simulink model "ES011A_DualEcuIdn"  (R2013b)
settings: Solver=FixedStepDiscrete  SolverMode=SingleTasking  StartTime=0.0  StopTime=1  FixedStep=0.002  RelTol=1e-3
values from neighbouring files (symbols this model uses):
  ECUCOMTIOUTFLT_CNT_U08 = DataDict.Constant    [ES011A_DualEcuIdn_DataDict.m]
  ECUID1_CNT_U08 = DataDict.Constant    [ES011A_DualEcuIdn_DataDict.m]
  ECUID2_CNT_U08 = DataDict.Constant    [ES011A_DualEcuIdn_DataDict.m]
  ECUIDINVLD_CNT_U08 = DataDict.Constant    [ES011A_DualEcuIdn_DataDict.m]
  IDENTCLECUIDNFLT_CNT_U08 = DataDict.Constant    [ES011A_DualEcuIdn_DataDict.m]
  IMCARBN_DUALECUIDNSECDRYECUIDN_CNT_U16 = DataDict.Constant    [ES011A_DualEcuIdn_DataDict.m]
  PRIMECUIDNOTREADFLT_CNT_U08 = DataDict.Constant    [ES011A_DualEcuIdn_DataDict.m]
  PRIMECUINVLDIDFLT_CNT_U08 = DataDict.Constant    [ES011A_DualEcuIdn_DataDict.m]
  SECDRYECUIDNOTREADFLT_CNT_U08 = DataDict.Constant    [ES011A_DualEcuIdn_DataDict.m]
  SECDRYECUIDNREQTIOUTVAL_CNT_U08 = DataDict.Constant    [ES011A_DualEcuIdn_DataDict.m]
  SECDRYECUINVLDIDFLT_CNT_U08 = DataDict.Constant    [ES011A_DualEcuIdn_DataDict.m]
  SECDRYECUREQIDTIOUTFLT_CNT_U08 = DataDict.Constant    [ES011A_DualEcuIdn_DataDict.m]
  VLDECUID_CNT_U08 = DataDict.Constant    [ES011A_DualEcuIdn_DataDict.m]
undefined symbols (not defined in the file or in its folder): NtcNr1, NtcSts1, sigbuilder_block
libraries: simulink x2
(part 1 of 2)
settings Model: Creator=cz68ds  LastModifiedBy=nzg49t
settings SolverCC: AutoInsertRateTranBlk=on  InsertRTBMode=Always
settings DataIOCC: LimitDataPoints=off  SaveFormat=Structure  ReturnWorkspaceOutputs=on
settings OptimizationCC: BlockReduction=off  InlineParams=on  ZeroExternalMemoryAtStartup=off  ZeroInternalMemoryAtStartup=off  OptimizeModelRefInitCode=on  LifeSpan=1
settings DebuggingCC: SignalInfNanChecking=error  SignalRangeChecking=warning  UnderspecifiedInitializationDetection=Simplified  SolverPrmCheckMsg=error  InheritedTsInSrcMsg=error  DiscreteInheritContinuousMsg=error  SingleTaskRateTransMsg=error  TasksWithSamePriorityMsg=error  SigSpecEnsureSampleTimeMsg=error  CheckMatrixSingularityMsg=error  ParameterUnderflowMsg=error  ParameterPrecisionLossMsg=error  ParameterTunabilityLossMsg=error  FixptConstUnderflowMsg=warning  FixptConstOverflowMsg=warning  VectorMatrixConversionMsg=error  SignalLabelMismatchMsg=error  UnconnectedInputMsg=error  UnconnectedOutputMsg=error  UnconnectedLineMsg=error  SFcnCompatibilityMsg=error  UniqueDataStoreMsg=warning  BusObjectLabelMismatch=error  RootOutportRequireBusObject=error  AssertControl=DisableAll  ModelReferenceIOMsg=error  ModelReferenceVersionMismatchMessage=warning  ModelReferenceIOMismatchMessage=error  ModelReferenceCSMismatchMessage=warning  ModelReferenceDataLoggingMessage=error  StateNameClashWarn=warning  StrictBusMsg=ErrorOnBusTreatedAsVector  NonBusSignalsTreatedAsBus=error  SFUnexpectedBacktrackingDiag=error  SFInvalidInputDataAccessInChartInitDiag=error  SFNoUnconditionalDefaultTransitionDiag=error  SFTransitionOutsideNaturalParentDiag=error  SFUnconditionalTransitionShadowingDiag=error  SFUndirectedBroadcastEventsDiag=error
settings ModelReferenceCC: ModelReferenceNumInstancesAllowed=Single
settings RTWCC: SystemTargetFile=autosar.tlc  GenCodeOnly=on  TemplateMakefile=ert_default_tmf  Description=AUTOSAR  GenerateReport=on  ProcessScript=autosar_make_rtw_hook  LaunchReport=on
settings CodeAppCC: GenerateComments=off  IgnoreCustomStorageClasses=off  CustomSymbolStrType=$N$R$M  CustomSymbolStrBlkIO=$N$M  SimulinkBlockComments=off
settings STFCustomTargetCC: ParMdlRefBuildCompliant=on  CompOptLevelCompliant=on  IncludeMdlTerminateFcn=off  CombineOutputUpdateFcns=on  SuppressErrorStatus=on  ERTFirstTimeCompliant=on  ERTCustomFileBanners=on  SupportNonFinite=off  SupportComplex=off  SupportContinuousTime=off  SupportNonInlinedSFcns=off  MATLABClassNameForMDSCustomization=Simulink.SoftwareTarget.ERTCustomization  AutosarCompliant=on  GRTInterface=off  SystemTargetFile=autosar.tlc
settings ERTTargetCC: CodeReplacementLibrary=ANSI_C  ConcurrentExecutionCompliant=off  IncludeMdlTerminateFcn=off  SuppressErrorStatus=on  SupportNonFinite=off  SupportComplex=off  ModelStepFunctionPrototypeControlCompliant=off  CPPClassGenCompliant=off  AutosarCompliant=on  InlinedParameterPlacement=NonHierarchical  ERTCustomFileTemplate=example_file_process.tlc  EnableUserReplacementTypes=on

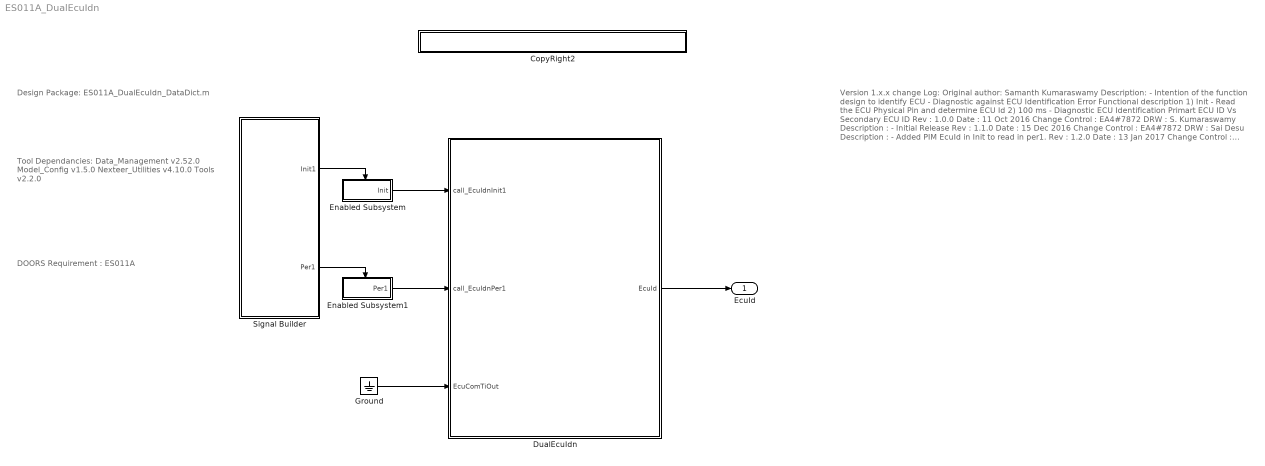
== system ES011A_DualEcuIdn ==
  note: Design Package:
      |
      | ES011A_DualEcuIdn_DataDict.m
  note: Tool Dependancies:
      |
      | Data_Management v2.52.0
      | Model_Config v1.5.0
      | Nexteer_Utilities v4.10.0
      | Tools v2.2.0
  note: DOORS Requirement :
      |
      | ES011A
  note: Version 1.x.x change Log:
      |
      | Original author: Samanth Kumaraswamy
      | Description:
      | - Intention of the function design to identify ECU
      | - Diagnostic against ECU Identification Error
      |
      | Functional description
      | 1) Init - Read the ECU Physical Pin and determine ECU Id
      | 2) 100 ms - Diagnostic ECU Identification Primart ECU ID Vs Secondary ECU ID
      |
      | Rev					: 1.0.0
      | Date					: 11 Oct 2016
      | Change Control		: EA4#7872
      | DRW					: S. Kumaraswamy
      | Description			:
      | - Initial Release
      |
      | Rev					: 1.1.0
      | Date					: 15 Dec 2016
      | Change Control		: EA4#7872
      | DRW					: Sai Desu
      | Description			:
      | - Added PIM EcuId in Init to read in per1.
      |
      | Rev					: 1.2.0
      | Date					: 13 Jan 2017
      | Change Control		: EA4#9279
      | DRW					: S. Kumaraswamy
      | Description			:
      | - Edited the PIM's name
      | - Added SetNtcSts in .m file as client call
  CopyRight2 : Subsystem  Description=|  mask(Copyright Information){none=on}
      | Copyright info block.                                               
      |                                                                     
      | Place copyright information at the top of every subsystem in design.
      mask prompts: none "No parameters"
      mask help: Place copyright information at the top of every subsystem in design.
      mask Display:
      | NxtrConf = 'Nexteer Confidential';
      | 
      | sys = bdroot; %handle for the current model ("system")
      | first = get_param(sys,'Created');
      | first = first(end-3:end);  %year is last four digits
      | 
      | last = get_param(sys,'LastModifiedDate');
      | if isempty(last)
      |     last = datestr(now,'yyyy');
      | else
      |     last = last(end-3:end);
      | end
      | 
      | if strcmp(first,last)
      |     fprintf('%s -- Copyright %s Nexteer',NxtrConf,first)
      | else
      |     fprintf('%s -- %s%s- %s Nexteer',NxtrConf,char(169),first,last)
      | end
  DualEcuIdn : Subsystem
  Enabled Subsystem : Subsystem  TreatAsAtomicUnit=on
  Enabled Subsystem1 : Subsystem  TreatAsAtomicUnit=on
  Ground : Ground
  Signal Builder : Subsystem  Tag=STV Subsys  LoadFcn=sigbuilder_block('load');  StartFcn=sigbuilder_block('start');  StopFcn=sigbuilder_block('stop');  ClipboardFcn=sigbuilder_block('clipboard');  mask(Sigbuilder block){}
      mask help: Simulink:masks:SigbuilderBlock_MD
      mask init:
      | if ~strcmp(get_param(bdroot(gcbh),'SimulationStatus'),'stopped') tuvar = sigbuilder_block('maskInit'); end
      settings: CopyFcn=sigbuilder_block('copy');  DeleteFcn=sigbuilder_block('delete');  ModelCloseFcn=sigbuilder_block('modelClose');  PreSaveFcn=sigbuilder_block('preSave');  PauseFcn=sigbuilder_block('pause');  ContinueFcn=sigbuilder_block('continue');  NameChangeFcn=sigbuilder_block('namechange');  OpenFcn=sigbuilder_block('open',[0 29.7931 1191.72 587.172 ]);  CloseFcn=sigbuilder_block('close');
      mask Display: plot(0, 0, 100, 100,[2, 2, 32, 32, 2], [68, 8, 8, 68, 68],[32, 2], [38, 38], [32, 19, 2],[53, 60, 44], [32, 17, 17, 2],[16, 16, 31, 31]);txt = getActiveGroup(gcbh);text(2, 100, txt,'verticalAlignment', 'top');
  EcuId : Outport
  wires:
  DualEcuIdn/1(EcuId) -> EcuId/1
  Enabled Subsystem/1(Init) -> DualEcuIdn/1(call_EcuIdnInit1)
  Ground/1 -> DualEcuIdn/3(EcuComTiOut)
  Signal Builder/1(Init1) -> Enabled Subsystem/Enable
  Enabled Subsystem1/1(Per1) -> DualEcuIdn/2(call_EcuIdnPer1)
  Signal Builder/2(Per1) -> Enabled Subsystem1/Enable

== system ES011A_DualEcuIdn/CopyRight2 ==

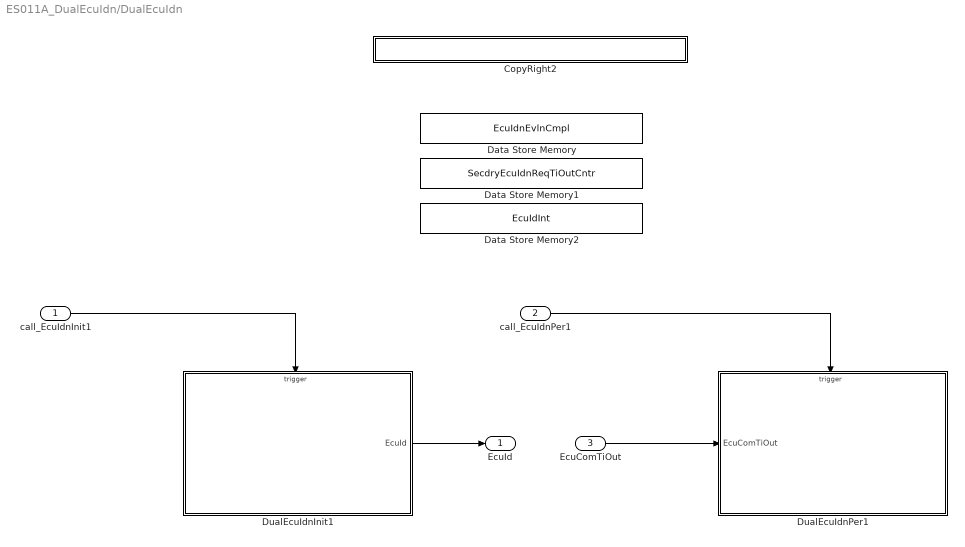
== system ES011A_DualEcuIdn/DualEcuIdn ==
  call_EcuIdnInit1 : Inport
  call_EcuIdnPer1 : Inport  Port=2
  EcuComTiOut : Inport  RequirementInfo={'linktype_rmi_doors' '00011b56 (/ESG Group/FDD Module Requirements/EA4 Specific/ES011A_DualEcuIdn)' '#ES011A_30' 'true' 'REQ:ES011A_30' '' } %GIDa_989c1e84_47d6_4077_a2ae_3e146373df7e  Port=3
  CopyRight2 : Subsystem  Description=|  mask(Copyright Information){none=on}
      | Copyright info block.                                               
      |                                                                     
      | Place copyright information at the top of every subsystem in design.
      mask prompts: none "No parameters"
      mask help: Place copyright information at the top of every subsystem in design.
      mask Display:
      | NxtrConf = 'Nexteer Confidential';
      | 
      | sys = bdroot; %handle for the current model ("system")
      | first = get_param(sys,'Created');
      | first = first(end-3:end);  %year is last four digits
      | 
      | last = get_param(sys,'LastModifiedDate');
      | if isempty(last)
      |     last = datestr(now,'yyyy');
      | else
      |     last = last(end-3:end);
      | end
      | 
      | if strcmp(first,last)
      |     fprintf('%s -- Copyright %s Nexteer',NxtrConf,first)
      | else
      |     fprintf('%s -- %s%s- %s Nexteer',NxtrConf,char(169),first,last)
      | end
  Data Store Memory : DataStoreMemory  DataStoreName=EcuIdnEvlnCmpl  OutDataTypeStr=boolean  StateMustResolveToSignalObject=on
  Data Store Memory1 : DataStoreMemory  DataStoreName=SecdryEcuIdnReqTiOutCntr  ReadBeforeWriteMsg=warning  WriteAfterWriteMsg=warning  WriteAfterReadMsg=warning  OutDataTypeStr=uint8  StateMustResolveToSignalObject=on
  Data Store Memory2 : DataStoreMemory  DataStoreName=EcuIdInt  OutDataTypeStr=uint8  StateMustResolveToSignalObject=on
  DualEcuIdnInit1 : Subsystem  RequirementInfo={'linktype_rmi_doors' '00011b56 (/ESG Group/FDD Module Requirements/EA4 Specific/ES011A_DualEcuIdn)' '#ES011A_56' 'true' 'REQ:ES011A_56' '' } %GIDa_248ec188_8c94_4ea4_99f3_45ec3f411dd5  TreatAsAtomicUnit=on
  DualEcuIdnPer1 : Subsystem  TreatAsAtomicUnit=on
  EcuId : Outport  RequirementInfo={'linktype_rmi_doors' '00011b56 (/ESG Group/FDD Module Requirements/EA4 Specific/ES011A_DualEcuIdn)' '#ES011A_31' 'true' 'REQ:ES011A_31' '' } %GIDa_18f308b4_0b0b_460d_b1e9_0f3a9849a141
  wires:
  call_EcuIdnInit1/1 -> DualEcuIdnInit1/Trigger
  call_EcuIdnPer1/1 -> DualEcuIdnPer1/Trigger
  DualEcuIdnInit1/1(EcuId) -> EcuId/1
  EcuComTiOut/1 -> DualEcuIdnPer1/1(EcuComTiOut)

== system ES011A_DualEcuIdn/Enabled Subsystem ==
  Enable : EnablePort
  Function Call Trigger2 : simulink/Ports & Subsystems/Function-Call Generator  RequirementInfo={} %GIDa_b8285886_6bd1_4885_ac08_252502d484ae  sample_time=0.1  numberOfIterations=1
      settings: AttributesFormatString=%<sample_time>
  Init : Outport
  wires:
  Function Call Trigger2/1 -> Init/1

== system ES011A_DualEcuIdn/Enabled Subsystem1 ==
  Enable : EnablePort
  Function Call Trigger1 : simulink/Ports & Subsystems/Function-Call Generator  RequirementInfo={} %GIDa_41275702_d4e5_428b_b5a8_ee66f9a793ef  sample_time=0.1  numberOfIterations=1
      settings: AttributesFormatString=%<sample_time>
  Per1 : Outport
  wires:
  Function Call Trigger1/1 -> Per1/1

== system ES011A_DualEcuIdn/Signal Builder ==
  Demux : Demux  Tag=STV Demux  Outputs=2
  FromWs : FromWorkspace  Tag=STV FromWs  VariableName=tuvar  SampleTime=0
      SigBuilderData=|
      | common.afterFinalStr = 'Extrapolate'
      | common.sampleTime = 0
      | dataSet.timeRange = [0 10]
      | dataSet.name = 'Group 1'
      | sbobj.Groups.Name = 'Group 1'
      | sbobj.Groups.Signals(1).Name = 'Init1'
      | sbobj.Groups.Signals(1).XData = [0 0.1 0.1 10]
      | sbobj.Groups.Signals(1).YData = [1 1 0 0]
      | sbobj.Groups.Signals(2).Name = 'Per1'
      | sbobj.Groups.Signals(2).XData = [0 0.1 0.1 10]
      | sbobj.Groups.Signals(2).YData = [0 0 1 1]
  Init1 : Outport  Tag=STV Outport
  Per1 : Outport  Tag=STV Outport  Port=2
  wires:
  Demux/1 -> Init1/1
  FromWs/1 -> Demux/1
  Demux/2 -> Per1/1

== system ES011A_DualEcuIdn/DualEcuIdn/CopyRight2 ==

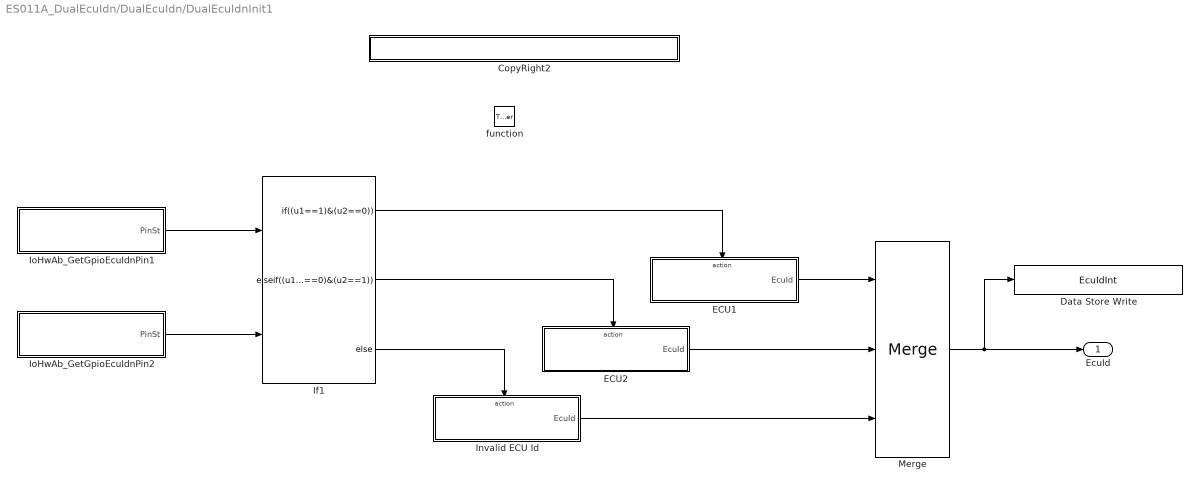
== system ES011A_DualEcuIdn/DualEcuIdn/DualEcuIdnInit1 ==
  function : TriggerPort  TriggerType=function-call
  CopyRight2 : Subsystem  Description=|  mask(Copyright Information){none=on}
      | Copyright info block.                                               
      |                                                                     
      | Place copyright information at the top of every subsystem in design.
      mask prompts: none "No parameters"
      mask help: Place copyright information at the top of every subsystem in design.
      mask Display:
      | NxtrConf = 'Nexteer Confidential';
      | 
      | sys = bdroot; %handle for the current model ("system")
      | first = get_param(sys,'Created');
      | first = first(end-3:end);  %year is last four digits
      | 
      | last = get_param(sys,'LastModifiedDate');
      | if isempty(last)
      |     last = datestr(now,'yyyy');
      | else
      |     last = last(end-3:end);
      | end
      | 
      | if strcmp(first,last)
      |     fprintf('%s -- Copyright %s Nexteer',NxtrConf,first)
      | else
      |     fprintf('%s -- %s%s- %s Nexteer',NxtrConf,char(169),first,last)
      | end
  Data Store Write : DataStoreWrite  DataStoreName=EcuIdInt
  ECU1 : Subsystem  TreatAsAtomicUnit=on
  ECU2 : Subsystem  TreatAsAtomicUnit=on
  If1 : If  NumInputs=2  IfExpression=(u1==1)&(u2==0)  ElseIfExpressions=(u1==0)&(u2==1)
  Invalid ECU Id : Subsystem  TreatAsAtomicUnit=on
  IoHwAb_GetGpioEcuIdnPin1 : Subsystem
  IoHwAb_GetGpioEcuIdnPin2 : Subsystem
  Merge : Merge  Inputs=3
  EcuId : Outport
  wires:
  Merge/1 -> Data Store Write/1, EcuId/1
  If1/1 -> ECU1/Action
  If1/3 -> Invalid ECU Id/Action
  ECU1/1(EcuId) -> Merge/1
  IoHwAb_GetGpioEcuIdnPin1/1(PinSt) -> If1/1
  Invalid ECU Id/1(EcuId) -> Merge/3
  IoHwAb_GetGpioEcuIdnPin2/1(PinSt) -> If1/2
  If1/2 -> ECU2/Action
  ECU2/1(EcuId) -> Merge/2

== system ES011A_DualEcuIdn/DualEcuIdn/DualEcuIdnPer1 ==
  EcuComTiOut : Inport
  function : TriggerPort  TriggerType=function-call
  CopyRight2 : Subsystem  Description=|  mask(Copyright Information){none=on}
      | Copyright info block.                                               
      |                                                                     
      | Place copyright information at the top of every subsystem in design.
      mask prompts: none "No parameters"
      mask help: Place copyright information at the top of every subsystem in design.
      mask Display:
      | NxtrConf = 'Nexteer Confidential';
      | 
      | sys = bdroot; %handle for the current model ("system")
      | first = get_param(sys,'Created');
      | first = first(end-3:end);  %year is last four digits
      | 
      | last = get_param(sys,'LastModifiedDate');
      | if isempty(last)
      |     last = datestr(now,'yyyy');
      | else
      |     last = last(end-3:end);
      | end
      | 
      | if strcmp(first,last)
      |     fprintf('%s -- Copyright %s Nexteer',NxtrConf,first)
      | else
      |     fprintf('%s -- %s%s- %s Nexteer',NxtrConf,char(169),first,last)
      | end
  Data Store Read : DataStoreRead  DataStoreName=EcuIdnEvlnCmpl
  Data Store Read1 : DataStoreRead  DataStoreName=EcuIdInt
  Evaluation Not Complete : Subsystem  TreatAsAtomicUnit=on
  If1 : If  IfExpression=u1 == 0  ShowElse=off
      settings: AttributesFormatString=|
      | %<IfExpression>
      | %<ElseIfExpressions>
  wires:
  Data Store Read/1 -> If1/1
  If1/1 -> Evaluation Not Complete/Action
  EcuComTiOut/1 -> Evaluation Not Complete/1(EcuComTiOut)
  Data Store Read1/1 -> Evaluation Not Complete/2(EcuIdn)

== system ES011A_DualEcuIdn/DualEcuIdn/DualEcuIdnInit1/CopyRight2 ==

== system ES011A_DualEcuIdn/DualEcuIdn/DualEcuIdnInit1/ECU1 ==
  Action Port : ActionPort  ActionType=then
  Constant : Constant  Value=ECUID1_CNT_U08
      settings: AttributesFormatString=%<Value>.EngVal = 1
  CopyRight2 : Subsystem  Description=|  mask(Copyright Information){none=on}
      | Copyright info block.                                               
      |                                                                     
      | Place copyright information at the top of every subsystem in design.
      mask prompts: none "No parameters"
      mask help: Place copyright information at the top of every subsystem in design.
      mask Display:
      | NxtrConf = 'Nexteer Confidential';
      | 
      | sys = bdroot; %handle for the current model ("system")
      | first = get_param(sys,'Created');
      | first = first(end-3:end);  %year is last four digits
      | 
      | last = get_param(sys,'LastModifiedDate');
      | if isempty(last)
      |     last = datestr(now,'yyyy');
      | else
      |     last = last(end-3:end);
      | end
      | 
      | if strcmp(first,last)
      |     fprintf('%s -- Copyright %s Nexteer',NxtrConf,first)
      | else
      |     fprintf('%s -- %s%s- %s Nexteer',NxtrConf,char(169),first,last)
      | end
  EcuId : Outport  InitialOutput=0
  wires:
  Constant/1 -> EcuId/1

== system ES011A_DualEcuIdn/DualEcuIdn/DualEcuIdnInit1/ECU2 ==
  Action Port : ActionPort  ActionType=elseif
  Constant : Constant  Value=ECUID2_CNT_U08
      settings: AttributesFormatString=%<Value>.EngVal = 2
  CopyRight2 : Subsystem  Description=|  mask(Copyright Information){none=on}
      | Copyright info block.                                               
      |                                                                     
      | Place copyright information at the top of every subsystem in design.
      mask prompts: none "No parameters"
      mask help: Place copyright information at the top of every subsystem in design.
      mask Display:
      | NxtrConf = 'Nexteer Confidential';
      | 
      | sys = bdroot; %handle for the current model ("system")
      | first = get_param(sys,'Created');
      | first = first(end-3:end);  %year is last four digits
      | 
      | last = get_param(sys,'LastModifiedDate');
      | if isempty(last)
      |     last = datestr(now,'yyyy');
      | else
      |     last = last(end-3:end);
      | end
      | 
      | if strcmp(first,last)
      |     fprintf('%s -- Copyright %s Nexteer',NxtrConf,first)
      | else
      |     fprintf('%s -- %s%s- %s Nexteer',NxtrConf,char(169),first,last)
      | end
  EcuId : Outport  InitialOutput=0
  wires:
  Constant/1 -> EcuId/1

== system ES011A_DualEcuIdn/DualEcuIdn/DualEcuIdnInit1/Invalid ECU Id ==
  Action Port : ActionPort  ActionType=else
  Constant2 : Constant  Value=ECUIDINVLD_CNT_U08
      settings: AttributesFormatString=%<Value>.EngVal = 3
  CopyRight2 : Subsystem  Description=|  mask(Copyright Information){none=on}
      | Copyright info block.                                               
      |                                                                     
      | Place copyright information at the top of every subsystem in design.
      mask prompts: none "No parameters"
      mask help: Place copyright information at the top of every subsystem in design.
      mask Display:
      | NxtrConf = 'Nexteer Confidential';
      | 
      | sys = bdroot; %handle for the current model ("system")
      | first = get_param(sys,'Created');
      | first = first(end-3:end);  %year is last four digits
      | 
      | last = get_param(sys,'LastModifiedDate');
      | if isempty(last)
      |     last = datestr(now,'yyyy');
      | else
      |     last = last(end-3:end);
      | end
      | 
      | if strcmp(first,last)
      |     fprintf('%s -- Copyright %s Nexteer',NxtrConf,first)
      | else
      |     fprintf('%s -- %s%s- %s Nexteer',NxtrConf,char(169),first,last)
      | end
  EcuId : Outport  InitialOutput=0
  wires:
  Constant2/1 -> EcuId/1

== system ES011A_DualEcuIdn/DualEcuIdn/DualEcuIdnInit1/IoHwAb_GetGpioEcuIdnPin1 ==
  CopyRight1 : Subsystem  Description=|  mask(Copyright Information){none=on}
      | Copyright info block.                                               
      |                                                                     
      | Place copyright information at the top of every subsystem in design.
      mask prompts: none "No parameters"
      mask help: Place copyright information at the top of every subsystem in design.
      mask Display:
      | NxtrConf = 'Nexteer Confidential';
      | 
      | sys = bdroot; %handle for the current model ("system")
      | first = get_param(sys,'Created');
      | first = first(end-3:end);  %year is last four digits
      | 
      | last = get_param(sys,'LastModifiedDate');
      | if isempty(last)
      |     last = datestr(now,'yyyy');
      | else
      |     last = last(end-3:end);
      | end
      | 
      | if strcmp(first,last)
      |     fprintf('%s -- Copyright %s Nexteer',NxtrConf,first)
      | else
      |     fprintf('%s -- %s%s- %s Nexteer',NxtrConf,char(169),first,last)
      | end
  Ground : Ground
  PinSt : Outport
  wires:
  Ground/1 -> PinSt/1

== system ES011A_DualEcuIdn/DualEcuIdn/DualEcuIdnInit1/IoHwAb_GetGpioEcuIdnPin2 ==
  CopyRight1 : Subsystem  Description=|  mask(Copyright Information){none=on}
      | Copyright info block.                                               
      |                                                                     
      | Place copyright information at the top of every subsystem in design.
      mask prompts: none "No parameters"
      mask help: Place copyright information at the top of every subsystem in design.
      mask Display:
      | NxtrConf = 'Nexteer Confidential';
      | 
      | sys = bdroot; %handle for the current model ("system")
      | first = get_param(sys,'Created');
      | first = first(end-3:end);  %year is last four digits
      | 
      | last = get_param(sys,'LastModifiedDate');
      | if isempty(last)
      |     last = datestr(now,'yyyy');
      | else
      |     last = last(end-3:end);
      | end
      | 
      | if strcmp(first,last)
      |     fprintf('%s -- Copyright %s Nexteer',NxtrConf,first)
      | else
      |     fprintf('%s -- %s%s- %s Nexteer',NxtrConf,char(169),first,last)
      | end
  Ground : Ground
  PinSt : Outport
  wires:
  Ground/1 -> PinSt/1

== system ES011A_DualEcuIdn/DualEcuIdn/DualEcuIdnPer1/CopyRight2 ==

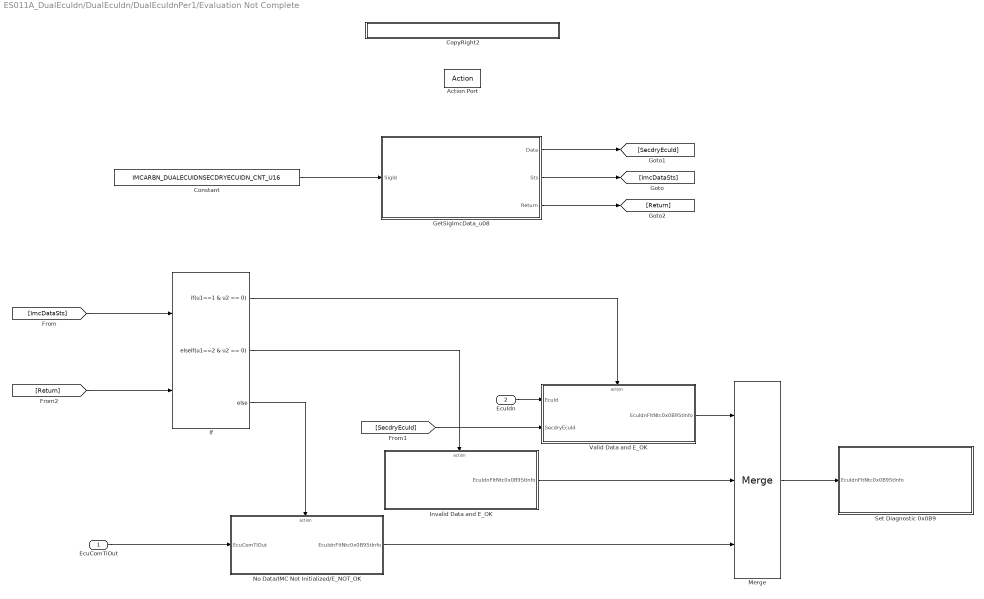
== system ES011A_DualEcuIdn/DualEcuIdn/DualEcuIdnPer1/Evaluation Not Complete ==
  EcuComTiOut : Inport
  EcuIdn : Inport  Port=2
  Action Port : ActionPort  ActionType=then
  Constant : Constant  Value=IMCARBN_DUALECUIDNSECDRYECUIDN_CNT_U16
  CopyRight2 : Subsystem  Description=|  mask(Copyright Information){none=on}
      | Copyright info block.                                               
      |                                                                     
      | Place copyright information at the top of every subsystem in design.
      mask prompts: none "No parameters"
      mask help: Place copyright information at the top of every subsystem in design.
      mask Display:
      | NxtrConf = 'Nexteer Confidential';
      | 
      | sys = bdroot; %handle for the current model ("system")
      | first = get_param(sys,'Created');
      | first = first(end-3:end);  %year is last four digits
      | 
      | last = get_param(sys,'LastModifiedDate');
      | if isempty(last)
      |     last = datestr(now,'yyyy');
      | else
      |     last = last(end-3:end);
      | end
      | 
      | if strcmp(first,last)
      |     fprintf('%s -- Copyright %s Nexteer',NxtrConf,first)
      | else
      |     fprintf('%s -- %s%s- %s Nexteer',NxtrConf,char(169),first,last)
      | end
  GetSigImcData_u08 : Subsystem  RequirementInfo={'linktype_rmi_doors' '00011b56 (/ESG Group/FDD Module Requirements/EA4 Specific/ES011A_DualEcuIdn)' '#ES011A_90' 'true' 'REQ:ES011A_90' '' } %GIDa_ed20b1a1_5e28_4aa9_88c9_d6d1ef14f358
  If : If  NumInputs=2  IfExpression=u1==1 & u2 == 0  ElseIfExpressions=u1==2 & u2 == 0
  Invalid Data and E_OK : Subsystem  RequirementInfo={'linktype_rmi_doors' '00011b56 (/ESG Group/FDD Module Requirements/EA4 Specific/ES011A_DualEcuIdn)' '#ES011A_91' 'true' 'REQ:ES011A_91' '' } %GIDa_1c1f80f6_7dca_4b27_9c6e_a34a3c8b287c  TreatAsAtomicUnit=on
  Merge : Merge  Inputs=3
  No Data/IMC Not Initialized/E_NOT_OK : Subsystem  RequirementInfo={'linktype_rmi_doors' '00011b56 (/ESG Group/FDD Module Requirements/EA4 Specific/ES011A_DualEcuIdn)' '#ES011A_97' 'true' 'REQ:ES011A_97' '' } %GIDa_2410bd0b_e67b_4f7b_b06c_d7360d71147d  TreatAsAtomicUnit=on
  Set Diagnostic 0x0B9 : Subsystem  RequirementInfo={'linktype_rmi_doors' '00011b56 (/ESG Group/FDD Module Requirements/EA4 Specific/ES011A_DualEcuIdn)' '#ES011A_83' 'true' 'REQ:ES011A_83' '' } %GIDa_fb7b3ce6_5e6d_4590_bdea_0a1abb4efd4c
  Valid Data and E_OK : Subsystem  TreatAsAtomicUnit=on
  wires:
  If/1 -> Valid Data and E_OK/Action
  If/3 -> No Data/IMC Not Initialized/E_NOT_OK/Action
  [SecdryEcuId] -> Valid Data and E_OK/2(SecdryEcuId)
  [ImcDataSts] -> If/1
  EcuComTiOut/1 -> No Data/IMC Not Initialized/E_NOT_OK/1(EcuComTiOut)
  If/2 -> Invalid Data and E_OK/Action
  EcuIdn/1 -> Valid Data and E_OK/1(EcuId)
  Valid Data and E_OK/1(EcuIdnFltNtc0x0B9StInfo) -> Merge/1
  Invalid Data and E_OK/1(EcuIdnFltNtc0x0B9StInfo) -> Merge/2
  No Data/IMC Not Initialized/E_NOT_OK/1(EcuIdnFltNtc0x0B9StInfo) -> Merge/3
  Constant/1 -> GetSigImcData_u08/1(SigId)
  GetSigImcData_u08/2(Sts) -> [ImcDataSts]
  GetSigImcData_u08/1(Data) -> [SecdryEcuId]
  GetSigImcData_u08/3(Return) -> [Return]
  [Return] -> If/2
  Merge/1 -> Set Diagnostic 0x0B9/1(EcuIdnFltNtc0x0B9StInfo)

== system ES011A_DualEcuIdn/DualEcuIdn/DualEcuIdnInit1/ECU1/CopyRight2 ==

== system ES011A_DualEcuIdn/DualEcuIdn/DualEcuIdnInit1/ECU2/CopyRight2 ==

== system ES011A_DualEcuIdn/DualEcuIdn/DualEcuIdnInit1/Invalid ECU Id/CopyRight2 ==

== system ES011A_DualEcuIdn/DualEcuIdn/DualEcuIdnInit1/IoHwAb_GetGpioEcuIdnPin1/CopyRight1 ==

== system ES011A_DualEcuIdn/DualEcuIdn/DualEcuIdnInit1/IoHwAb_GetGpioEcuIdnPin2/CopyRight1 ==

== system ES011A_DualEcuIdn/DualEcuIdn/DualEcuIdnPer1/Evaluation Not Complete/CopyRight2 ==

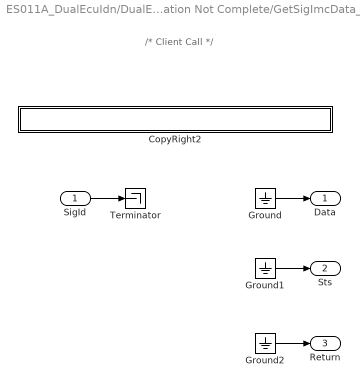
== system ES011A_DualEcuIdn/DualEcuIdn/DualEcuIdnPer1/Evaluation Not Complete/GetSigImcData_u08 ==
  note: /* Client Call */
  SigId : Inport
  CopyRight2 : Subsystem  Description=|  mask(Copyright Information){none=on}
      | Copyright info block.                                               
      |                                                                     
      | Place copyright information at the top of every subsystem in design.
      mask prompts: none "No parameters"
      mask help: Place copyright information at the top of every subsystem in design.
      mask Display:
      | NxtrConf = 'Nexteer Confidential';
      | 
      | sys = bdroot; %handle for the current model ("system")
      | first = get_param(sys,'Created');
      | first = first(end-3:end);  %year is last four digits
      | 
      | last = get_param(sys,'LastModifiedDate');
      | if isempty(last)
      |     last = datestr(now,'yyyy');
      | else
      |     last = last(end-3:end);
      | end
      | 
      | if strcmp(first,last)
      |     fprintf('%s -- Copyright %s Nexteer',NxtrConf,first)
      | else
      |     fprintf('%s -- %s%s- %s Nexteer',NxtrConf,char(169),first,last)
      | end
  Ground : Ground
  Ground1 : Ground
  Ground2 : Ground
  Terminator : Terminator
  Data : Outport
  Sts : Outport  Port=2
  Return : Outport  Port=3
  wires:
  SigId/1 -> Terminator/1
  Ground/1 -> Data/1
  Ground1/1 -> Sts/1
  Ground2/1 -> Return/1

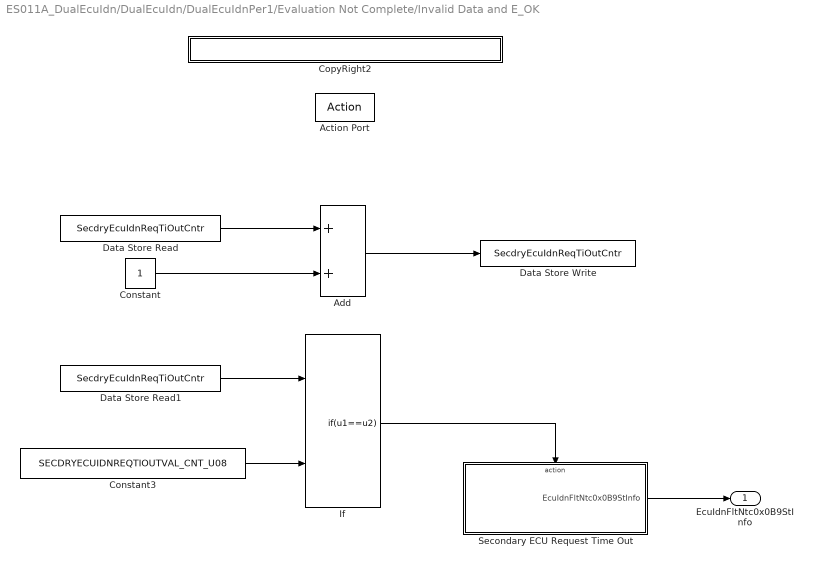
== system ES011A_DualEcuIdn/DualEcuIdn/DualEcuIdnPer1/Evaluation Not Complete/Invalid Data and E_OK ==
  Action Port : ActionPort  ActionType=elseif
  Add : Sum
  Constant : Constant  OutDataTypeStr=boolean
  Constant3 : Constant  Value=SECDRYECUIDNREQTIOUTVAL_CNT_U08
      settings: AttributesFormatString=%<Value>.EngVal = 10
  CopyRight2 : Subsystem  Description=|  mask(Copyright Information){none=on}
      | Copyright info block.                                               
      |                                                                     
      | Place copyright information at the top of every subsystem in design.
      mask prompts: none "No parameters"
      mask help: Place copyright information at the top of every subsystem in design.
      mask Display:
      | NxtrConf = 'Nexteer Confidential';
      | 
      | sys = bdroot; %handle for the current model ("system")
      | first = get_param(sys,'Created');
      | first = first(end-3:end);  %year is last four digits
      | 
      | last = get_param(sys,'LastModifiedDate');
      | if isempty(last)
      |     last = datestr(now,'yyyy');
      | else
      |     last = last(end-3:end);
      | end
      | 
      | if strcmp(first,last)
      |     fprintf('%s -- Copyright %s Nexteer',NxtrConf,first)
      | else
      |     fprintf('%s -- %s%s- %s Nexteer',NxtrConf,char(169),first,last)
      | end
  Data Store Read : DataStoreRead  DataStoreName=SecdryEcuIdnReqTiOutCntr
  Data Store Read1 : DataStoreRead  DataStoreName=SecdryEcuIdnReqTiOutCntr
  Data Store Write : DataStoreWrite  DataStoreName=SecdryEcuIdnReqTiOutCntr
  If : If  NumInputs=2  IfExpression=u1==u2  ShowElse=off
      settings: AttributesFormatString=|
      | %<IfExpression>
      | %<ElseIfExpressions>
  Secondary ECU Request Time Out : Subsystem  TreatAsAtomicUnit=on
  EcuIdnFltNtc0x0B9StInfo : Outport
  wires:
  Constant/1 -> Add/2
  Data Store Read/1 -> Add/1
  Add/1 -> Data Store Write/1
  Data Store Read1/1 -> If/1
  If/1 -> Secondary ECU Request Time Out/Action
  Secondary ECU Request Time Out/1(EcuIdnFltNtc0x0B9StInfo) -> EcuIdnFltNtc0x0B9StInfo/1
  Constant3/1 -> If/2

== system ES011A_DualEcuIdn/DualEcuIdn/DualEcuIdnPer1/Evaluation Not Complete/No Data//IMC Not Initialized//E_NOT_OK ==
  EcuComTiOut : Inport
  Action Port : ActionPort  ActionType=else
  CopyRight2 : Subsystem  Description=|  mask(Copyright Information){none=on}
      | Copyright info block.                                               
      |                                                                     
      | Place copyright information at the top of every subsystem in design.
      mask prompts: none "No parameters"
      mask help: Place copyright information at the top of every subsystem in design.
      mask Display:
      | NxtrConf = 'Nexteer Confidential';
      | 
      | sys = bdroot; %handle for the current model ("system")
      | first = get_param(sys,'Created');
      | first = first(end-3:end);  %year is last four digits
      | 
      | last = get_param(sys,'LastModifiedDate');
      | if isempty(last)
      |     last = datestr(now,'yyyy');
      | else
      |     last = last(end-3:end);
      | end
      | 
      | if strcmp(first,last)
      |     fprintf('%s -- Copyright %s Nexteer',NxtrConf,first)
      | else
      |     fprintf('%s -- %s%s- %s Nexteer',NxtrConf,char(169),first,last)
      | end
  ECU Communication Time Out : Subsystem  TreatAsAtomicUnit=on
  If : If  IfExpression=u1  ShowElse=off
      settings: AttributesFormatString=|
      | %<IfExpression>
      | %<ElseIfExpressions>
  EcuIdnFltNtc0x0B9StInfo : Outport
  wires:
  EcuComTiOut/1 -> If/1
  If/1 -> ECU Communication Time Out/Action
  ECU Communication Time Out/1(EcuIdnFltNtc0x0B9StInfo) -> EcuIdnFltNtc0x0B9StInfo/1

== system ES011A_DualEcuIdn/DualEcuIdn/DualEcuIdnPer1/Evaluation Not Complete/Set Diagnostic 0x0B9 ==
  EcuIdnFltNtc0x0B9StInfo : Inport
  CopyRight2 : Subsystem  Description=|  mask(Copyright Information){none=on}
      | Copyright info block.                                               
      |                                                                     
      | Place copyright information at the top of every subsystem in design.
      mask prompts: none "No parameters"
      mask help: Place copyright information at the top of every subsystem in design.
      mask Display:
      | NxtrConf = 'Nexteer Confidential';
      | 
      | sys = bdroot; %handle for the current model ("system")
      | first = get_param(sys,'Created');
      | first = first(end-3:end);  %year is last four digits
      | 
      | last = get_param(sys,'LastModifiedDate');
      | if isempty(last)
      |     last = datestr(now,'yyyy');
      | else
      |     last = last(end-3:end);
      | end
      | 
      | if strcmp(first,last)
      |     fprintf('%s -- Copyright %s Nexteer',NxtrConf,first)
      | else
      |     fprintf('%s -- %s%s- %s Nexteer',NxtrConf,char(169),first,last)
      | end
  Fail NTC : Subsystem  RequirementInfo={'linktype_rmi_doors' '00011b56 (/ESG Group/FDD Module Requirements/EA4 Specific/ES011A_DualEcuIdn)' '#ES011A_85' 'true' 'REQ:ES011A_85' '' ; 'linktype_rmi_doors' '00011b56 (/ESG Group/FDD Module Requirements/EA4 Specific/ES011A_DualEcuIdn)' '#ES011A_87' 'true' 'REQ:ES011A_87' '' ; 'linktype_rmi_doors' '00011b56 (/ESG Group/FDD Module Requirements/EA4 Specific/ES011A_DualEcuIdn)' '#ES011A_93' 'true' 'REQ:ES011A_93' '' } %GIDa_fcb7f1b1_36da_4613_beed_269da419cb1d  TreatAsAtomicUnit=on
  If1 : If  IfExpression=u1
  Pass NTC : Subsystem  RequirementInfo={'linktype_rmi_doors' '00011b56 (/ESG Group/FDD Module Requirements/EA4 Specific/ES011A_DualEcuIdn)' '#ES011A_84' 'true' 'REQ:ES011A_84' '' } %GIDa_e9a9345d_e238_4be2_9e8d_00234925b14a  TreatAsAtomicUnit=on
  wires:
  EcuIdnFltNtc0x0B9StInfo/1 -> If1/1, Pass NTC/1(EcuIdnFltNtc0x0B9StInfo), Fail NTC/1(EcuIdnFltNtc0x0B9StInfo)
  If1/1 -> Fail NTC/Action
  If1/2 -> Pass NTC/Action

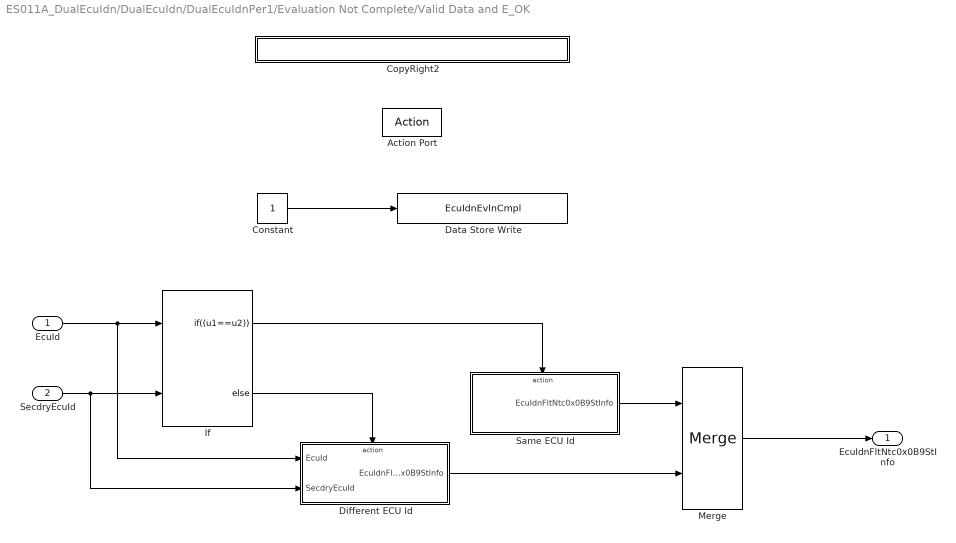
== system ES011A_DualEcuIdn/DualEcuIdn/DualEcuIdnPer1/Evaluation Not Complete/Valid Data and E_OK ==
  EcuId : Inport
  SecdryEcuId : Inport  Port=2
  Action Port : ActionPort  ActionType=then
  Constant : Constant  Description=TRUE  OutDataTypeStr=boolean
      settings: AttributesFormatString=TRUE
  CopyRight2 : Subsystem  Description=|  mask(Copyright Information){none=on}
      | Copyright info block.                                               
      |                                                                     
      | Place copyright information at the top of every subsystem in design.
      mask prompts: none "No parameters"
      mask help: Place copyright information at the top of every subsystem in design.
      mask Display:
      | NxtrConf = 'Nexteer Confidential';
      | 
      | sys = bdroot; %handle for the current model ("system")
      | first = get_param(sys,'Created');
      | first = first(end-3:end);  %year is last four digits
      | 
      | last = get_param(sys,'LastModifiedDate');
      | if isempty(last)
      |     last = datestr(now,'yyyy');
      | else
      |     last = last(end-3:end);
      | end
      | 
      | if strcmp(first,last)
      |     fprintf('%s -- Copyright %s Nexteer',NxtrConf,first)
      | else
      |     fprintf('%s -- %s%s- %s Nexteer',NxtrConf,char(169),first,last)
      | end
  Data Store Write : DataStoreWrite  DataStoreName=EcuIdnEvlnCmpl
  Different ECU Id : Subsystem  RequirementInfo={'linktype_rmi_doors' '00011b56 (/ESG Group/FDD Module Requirements/EA4 Specific/ES011A_DualEcuIdn)' '#ES011A_85' 'true' 'REQ:ES011A_85' '' ; 'linktype_rmi_doors' '00011b56 (/ESG Group/FDD Module Requirements/EA4 Specific/ES011A_DualEcuIdn)' '#ES011A_87' 'true' 'REQ:ES011A_87' '' ; 'linktype_rmi_doors' '00011b56 (/ESG Group/FDD Module Requirements/EA4 Specific/ES011A_DualEcuIdn)' '#ES011A_93' 'true' 'REQ:ES011A_93' '' } %GIDa_9aa029ba_03fe_4934_b810_1eaf33d1025b  TreatAsAtomicUnit=on
  If : If  NumInputs=2  IfExpression=(u1==u2)
  Merge : Merge
  Same ECU Id : Subsystem  RequirementInfo={'linktype_rmi_doors' '00011b56 (/ESG Group/FDD Module Requirements/EA4 Specific/ES011A_DualEcuIdn)' '#ES011A_98' 'true' 'REQ:ES011A_98' '' } %GIDa_85da6f46_22a2_458b_808d_fb46cf689a98  TreatAsAtomicUnit=on
  EcuIdnFltNtc0x0B9StInfo : Outport  InitialOutput=0
  wires:
  EcuId/1 -> Different ECU Id/1(EcuId), If/1
  SecdryEcuId/1 -> Different ECU Id/2(SecdryEcuId), If/2
  If/1 -> Same ECU Id/Action
  If/2 -> Different ECU Id/Action
  Same ECU Id/1(EcuIdnFltNtc0x0B9StInfo) -> Merge/1
  Different ECU Id/1(EcuIdnFltNtc0x0B9StInfo) -> Merge/2
  Constant/1 -> Data Store Write/1
  Merge/1 -> EcuIdnFltNtc0x0B9StInfo/1

== system ES011A_DualEcuIdn/DualEcuIdn/DualEcuIdnPer1/Evaluation Not Complete/GetSigImcData_u08/CopyRight2 ==

== system ES011A_DualEcuIdn/DualEcuIdn/DualEcuIdnPer1/Evaluation Not Complete/Invalid Data and E_OK/CopyRight2 ==

== system ES011A_DualEcuIdn/DualEcuIdn/DualEcuIdnPer1/Evaluation Not Complete/Invalid Data and E_OK/Secondary ECU Request Time Out ==
  Action Port : ActionPort  ActionType=then
  Constant1 : Constant  OutDataTypeStr=boolean
      settings: AttributesFormatString=TRUE
  Constant2 : Constant  Value=SECDRYECUREQIDTIOUTFLT_CNT_U08
      settings: AttributesFormatString=%<Value>.EngVal = 32
  CopyRight2 : Subsystem  Description=|  mask(Copyright Information){none=on}
      | Copyright info block.                                               
      |                                                                     
      | Place copyright information at the top of every subsystem in design.
      mask prompts: none "No parameters"
      mask help: Place copyright information at the top of every subsystem in design.
      mask Display:
      | NxtrConf = 'Nexteer Confidential';
      | 
      | sys = bdroot; %handle for the current model ("system")
      | first = get_param(sys,'Created');
      | first = first(end-3:end);  %year is last four digits
      | 
      | last = get_param(sys,'LastModifiedDate');
      | if isempty(last)
      |     last = datestr(now,'yyyy');
      | else
      |     last = last(end-3:end);
      | end
      | 
      | if strcmp(first,last)
      |     fprintf('%s -- Copyright %s Nexteer',NxtrConf,first)
      | else
      |     fprintf('%s -- %s%s- %s Nexteer',NxtrConf,char(169),first,last)
      | end
  Data Store Write1 : DataStoreWrite  DataStoreName=EcuIdnEvlnCmpl
  EcuIdnFltNtc0x0B9StInfo : Outport  InitialOutput=0
  wires:
  Constant1/1 -> Data Store Write1/1
  Constant2/1 -> EcuIdnFltNtc0x0B9StInfo/1

== system ES011A_DualEcuIdn/DualEcuIdn/DualEcuIdnPer1/Evaluation Not Complete/No Data//IMC Not Initialized//E_NOT_OK/CopyRight2 ==

== system ES011A_DualEcuIdn/DualEcuIdn/DualEcuIdnPer1/Evaluation Not Complete/No Data//IMC Not Initialized//E_NOT_OK/ECU Communication Time Out ==
  Action Port : ActionPort  ActionType=then
  Constant : Constant  OutDataTypeStr=boolean
      settings: AttributesFormatString=TRUE
  Constant2 : Constant  Value=ECUCOMTIOUTFLT_CNT_U08
      settings: AttributesFormatString=%<Value>.EngVal = 64
  CopyRight2 : Subsystem  Description=|  mask(Copyright Information){none=on}
      | Copyright info block.                                               
      |                                                                     
      | Place copyright information at the top of every subsystem in design.
      mask prompts: none "No parameters"
      mask help: Place copyright information at the top of every subsystem in design.
      mask Display:
      | NxtrConf = 'Nexteer Confidential';
      | 
      | sys = bdroot; %handle for the current model ("system")
      | first = get_param(sys,'Created');
      | first = first(end-3:end);  %year is last four digits
      | 
      | last = get_param(sys,'LastModifiedDate');
      | if isempty(last)
      |     last = datestr(now,'yyyy');
      | else
      |     last = last(end-3:end);
      | end
      | 
      | if strcmp(first,last)
      |     fprintf('%s -- Copyright %s Nexteer',NxtrConf,first)
      | else
      |     fprintf('%s -- %s%s- %s Nexteer',NxtrConf,char(169),first,last)
      | end
  Data Store Write : DataStoreWrite  DataStoreName=EcuIdnEvlnCmpl
  EcuIdnFltNtc0x0B9StInfo : Outport  InitialOutput=0
  wires:
  Constant/1 -> Data Store Write/1
  Constant2/1 -> EcuIdnFltNtc0x0B9StInfo/1

== system ES011A_DualEcuIdn/DualEcuIdn/DualEcuIdnPer1/Evaluation Not Complete/Set Diagnostic 0x0B9/CopyRight2 ==

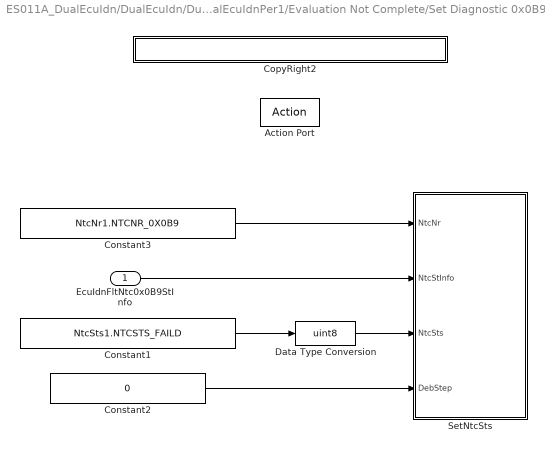
== system ES011A_DualEcuIdn/DualEcuIdn/DualEcuIdnPer1/Evaluation Not Complete/Set Diagnostic 0x0B9/Fail NTC ==
  EcuIdnFltNtc0x0B9StInfo : Inport
  Action Port : ActionPort  ActionType=then
  Constant1 : Constant  Value=NtcSts1.NTCSTS_FAILD
      settings: AttributesFormatString=%<Value> = 1
  Constant2 : Constant  Value=0  OutDataTypeStr=uint16
      settings: AttributesFormatString=0 Debounce Step
  Constant3 : Constant  Value=NtcNr1.NTCNR_0X0B9
  CopyRight2 : Subsystem  Description=|  mask(Copyright Information){none=on}
      | Copyright info block.                                               
      |                                                                     
      | Place copyright information at the top of every subsystem in design.
      mask prompts: none "No parameters"
      mask help: Place copyright information at the top of every subsystem in design.
      mask Display:
      | NxtrConf = 'Nexteer Confidential';
      | 
      | sys = bdroot; %handle for the current model ("system")
      | first = get_param(sys,'Created');
      | first = first(end-3:end);  %year is last four digits
      | 
      | last = get_param(sys,'LastModifiedDate');
      | if isempty(last)
      |     last = datestr(now,'yyyy');
      | else
      |     last = last(end-3:end);
      | end
      | 
      | if strcmp(first,last)
      |     fprintf('%s -- Copyright %s Nexteer',NxtrConf,first)
      | else
      |     fprintf('%s -- %s%s- %s Nexteer',NxtrConf,char(169),first,last)
      | end
  Data Type Conversion : DataTypeConversion  OutDataTypeStr=uint8
  SetNtcSts : Subsystem  RequirementInfo={} %GIDa_3a182333_0d11_4396_8898_32ca73e229d0
  wires:
  Constant1/1 -> Data Type Conversion/1
  Constant3/1 -> SetNtcSts/1(NtcNr)
  Constant2/1 -> SetNtcSts/4(DebStep)
  EcuIdnFltNtc0x0B9StInfo/1 -> SetNtcSts/2(NtcStInfo)
  Data Type Conversion/1 -> SetNtcSts/3(NtcSts)

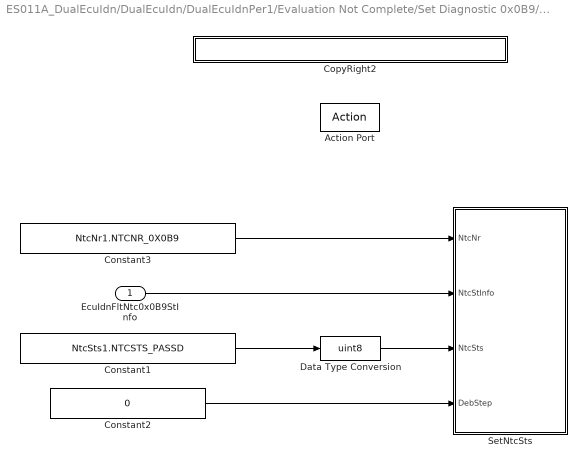
== system ES011A_DualEcuIdn/DualEcuIdn/DualEcuIdnPer1/Evaluation Not Complete/Set Diagnostic 0x0B9/Pass NTC ==
  EcuIdnFltNtc0x0B9StInfo : Inport
  Action Port : ActionPort  ActionType=else
  Constant1 : Constant  Value=NtcSts1.NTCSTS_PASSD
      settings: AttributesFormatString=%<Value> = 0
  Constant2 : Constant  Value=0  OutDataTypeStr=uint16
      settings: AttributesFormatString=0 Debounce Step
  Constant3 : Constant  Value=NtcNr1.NTCNR_0X0B9
  CopyRight2 : Subsystem  Description=|  mask(Copyright Information){none=on}
      | Copyright info block.                                               
      |                                                                     
      | Place copyright information at the top of every subsystem in design.
      mask prompts: none "No parameters"
      mask help: Place copyright information at the top of every subsystem in design.
      mask Display:
      | NxtrConf = 'Nexteer Confidential';
      | 
      | sys = bdroot; %handle for the current model ("system")
      | first = get_param(sys,'Created');
      | first = first(end-3:end);  %year is last four digits
      | 
      | last = get_param(sys,'LastModifiedDate');
      | if isempty(last)
      |     last = datestr(now,'yyyy');
      | else
      |     last = last(end-3:end);
      | end
      | 
      | if strcmp(first,last)
      |     fprintf('%s -- Copyright %s Nexteer',NxtrConf,first)
      | else
      |     fprintf('%s -- %s%s- %s Nexteer',NxtrConf,char(169),first,last)
      | end
  Data Type Conversion : DataTypeConversion  OutDataTypeStr=uint8
  SetNtcSts : Subsystem  RequirementInfo={} %GIDa_78d8682d_96e3_4ca0_bd38_167f9167f64c
  wires:
  Constant1/1 -> Data Type Conversion/1
  Constant3/1 -> SetNtcSts/1(NtcNr)
  Constant2/1 -> SetNtcSts/4(DebStep)
  EcuIdnFltNtc0x0B9StInfo/1 -> SetNtcSts/2(NtcStInfo)
  Data Type Conversion/1 -> SetNtcSts/3(NtcSts)

== system ES011A_DualEcuIdn/DualEcuIdn/DualEcuIdnPer1/Evaluation Not Complete/Valid Data and E_OK/CopyRight2 ==

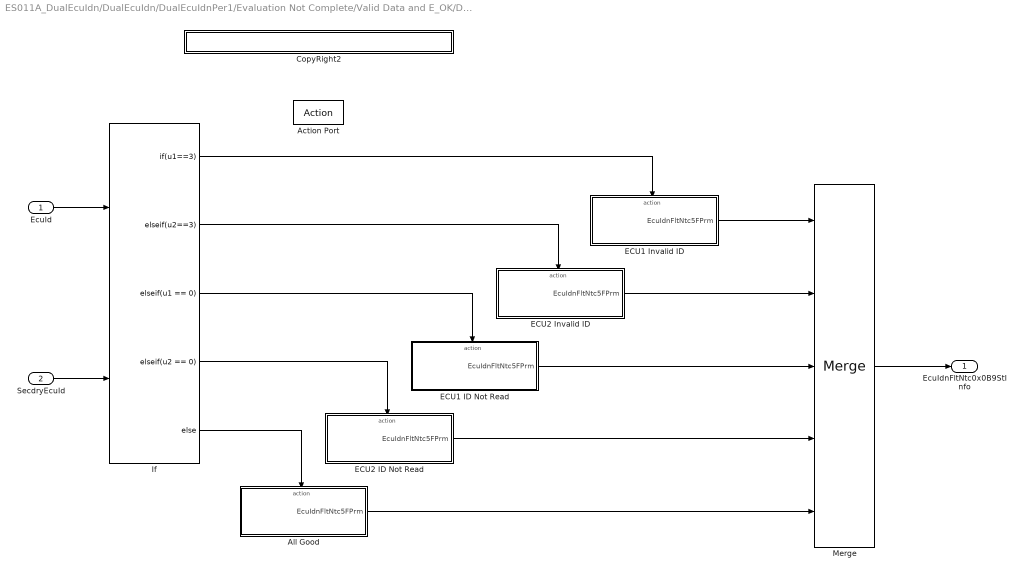
== system ES011A_DualEcuIdn/DualEcuIdn/DualEcuIdnPer1/Evaluation Not Complete/Valid Data and E_OK/Different ECU Id ==
  EcuId : Inport
  SecdryEcuId : Inport  Port=2
  Action Port : ActionPort  ActionType=else
  All Good : Subsystem  TreatAsAtomicUnit=on
  CopyRight2 : Subsystem  Description=|  mask(Copyright Information){none=on}
      | Copyright info block.                                               
      |                                                                     
      | Place copyright information at the top of every subsystem in design.
      mask prompts: none "No parameters"
      mask help: Place copyright information at the top of every subsystem in design.
      mask Display:
      | NxtrConf = 'Nexteer Confidential';
      | 
      | sys = bdroot; %handle for the current model ("system")
      | first = get_param(sys,'Created');
      | first = first(end-3:end);  %year is last four digits
      | 
      | last = get_param(sys,'LastModifiedDate');
      | if isempty(last)
      |     last = datestr(now,'yyyy');
      | else
      |     last = last(end-3:end);
      | end
      | 
      | if strcmp(first,last)
      |     fprintf('%s -- Copyright %s Nexteer',NxtrConf,first)
      | else
      |     fprintf('%s -- %s%s- %s Nexteer',NxtrConf,char(169),first,last)
      | end
  ECU1 ID Not Read : Subsystem  TreatAsAtomicUnit=on
  ECU1 Invalid ID : Subsystem  TreatAsAtomicUnit=on
  ECU2 ID Not Read : Subsystem  TreatAsAtomicUnit=on
  ECU2 Invalid ID : Subsystem  TreatAsAtomicUnit=on
  If : If  NumInputs=2  IfExpression=u1==3  ElseIfExpressions=u2==3, u1 == 0, u2 == 0
  Merge : Merge  Inputs=5
  EcuIdnFltNtc0x0B9StInfo : Outport  InitialOutput=0
  wires:
  EcuId/1 -> If/1
  SecdryEcuId/1 -> If/2
  If/1 -> ECU1 Invalid ID/Action
  If/2 -> ECU2 Invalid ID/Action
  If/5 -> All Good/Action
  ECU1 Invalid ID/1(EcuIdnFltNtc5FPrm) -> Merge/1
  ECU2 Invalid ID/1(EcuIdnFltNtc5FPrm) -> Merge/2
  Merge/1 -> EcuIdnFltNtc0x0B9StInfo/1
  If/4 -> ECU2 ID Not Read/Action
  If/3 -> ECU1 ID Not Read/Action
  ECU1 ID Not Read/1(EcuIdnFltNtc5FPrm) -> Merge/3
  ECU2 ID Not Read/1(EcuIdnFltNtc5FPrm) -> Merge/4
  All Good/1(EcuIdnFltNtc5FPrm) -> Merge/5

== system ES011A_DualEcuIdn/DualEcuIdn/DualEcuIdnPer1/Evaluation Not Complete/Valid Data and E_OK/Same ECU Id ==
  Action Port : ActionPort  ActionType=then
  CopyRight2 : Subsystem  Description=|  mask(Copyright Information){none=on}
      | Copyright info block.                                               
      |                                                                     
      | Place copyright information at the top of every subsystem in design.
      mask prompts: none "No parameters"
      mask help: Place copyright information at the top of every subsystem in design.
      mask Display:
      | NxtrConf = 'Nexteer Confidential';
      | 
      | sys = bdroot; %handle for the current model ("system")
      | first = get_param(sys,'Created');
      | first = first(end-3:end);  %year is last four digits
      | 
      | last = get_param(sys,'LastModifiedDate');
      | if isempty(last)
      |     last = datestr(now,'yyyy');
      | else
      |     last = last(end-3:end);
      | end
      | 
      | if strcmp(first,last)
      |     fprintf('%s -- Copyright %s Nexteer',NxtrConf,first)
      | else
      |     fprintf('%s -- %s%s- %s Nexteer',NxtrConf,char(169),first,last)
      | end
  Identical ECU Identification Fault Value = 1 : Constant  Value=IDENTCLECUIDNFLT_CNT_U08
  EcuIdnFltNtc0x0B9StInfo : Outport  InitialOutput=0
  wires:
  Identical ECU Identification Fault Value = 1/1 -> EcuIdnFltNtc0x0B9StInfo/1

== system ES011A_DualEcuIdn/DualEcuIdn/DualEcuIdnPer1/Evaluation Not Complete/Invalid Data and E_OK/Secondary ECU Request Time Out/CopyRight2 ==

== system ES011A_DualEcuIdn/DualEcuIdn/DualEcuIdnPer1/Evaluation Not Complete/No Data//IMC Not Initialized//E_NOT_OK/ECU Communication Time Out/CopyRight2 ==

== system ES011A_DualEcuIdn/DualEcuIdn/DualEcuIdnPer1/Evaluation Not Complete/Set Diagnostic 0x0B9/Fail NTC/CopyRight2 ==

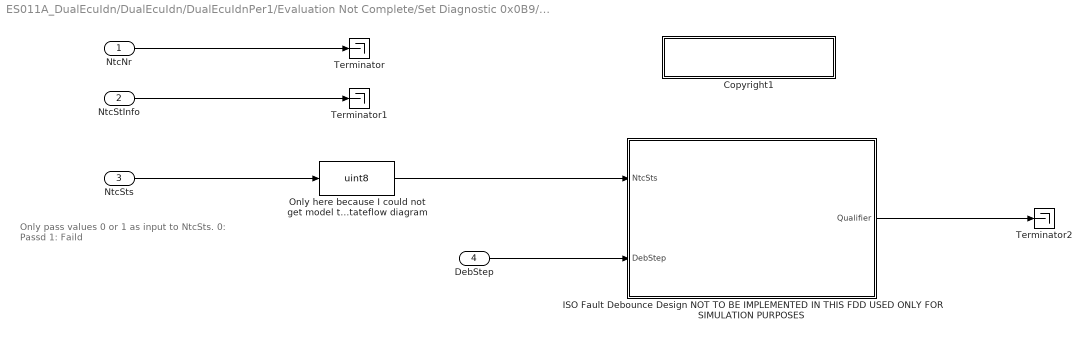
== system ES011A_DualEcuIdn/DualEcuIdn/DualEcuIdnPer1/Evaluation Not Complete/Set Diagnostic 0x0B9/Fail NTC/SetNtcSts ==
  note: Only pass values 0 or 1 as input to NtcSts.
      | 0: Passd
      | 1: Faild
  NtcNr : Inport
  NtcStInfo : Inport  Port=2
  NtcSts : Inport  Port=3  OutDataTypeStr=uint8
  DebStep : Inport  Port=4  OutDataTypeStr=uint16
  Copyright1 : Subsystem  Description=|  mask(Copyright Information){none=on}
      | Copyright info block.                                               
      |                                                                     
      | Place copyright information at the top of every subsystem in design.
      mask prompts: none "No parameters"
      mask help: Place copyright information at the top of every subsystem in design.
      mask Display:
      | NxtrConf = 'Nexteer Confidential';
      | 
      | sys = bdroot; %handle for the current model ("system")
      | first = get_param(sys,'Created');
      | if(isempty(first))
      |     first = datestr(now,'yyyy');
      | else
      |     first = first(end-3:end);  %year is last four digits
      | end
      | 
      | last = get_param(sys,'LastModifiedDate');
      | if isempty(last)
      |     last = datestr(now,'yyyy');
      | else
      |     last = last(end-3:end);
      | end
      | 
      | if strcmp(first,last)
      |     fprintf('%s\nCopyright  %s Nexteer',NxtrConf,first);
      | else
      |     fprintf('%s\n%s%s-%s Nexteer',NxtrConf,char(169),first,last);
      | end
  ISO Fault Debounce Design NOT TO BE IMPLEMENTED IN THIS FDD USED ONLY FOR SIMULATION PURPOSES : Stateflow chart  TreatAsAtomicUnit=on
  Only here because I could not get model to run with enumerations in the stateflow diagram : DataTypeConversion  OutDataTypeStr=uint8
  Terminator : Terminator
  Terminator1 : Terminator
  Terminator2 : Terminator
  wires:
  NtcStInfo/1 -> Terminator1/1
  NtcNr/1 -> Terminator/1
  NtcSts/1 -> Only here because I could not get model to run with enumerations in the stateflow diagram/1
  DebStep/1 -> ISO Fault Debounce Design NOT TO BE IMPLEMENTED IN THIS FDD USED ONLY FOR SIMULATION PURPOSES/2(DebStep)
  ISO Fault Debounce Design NOT TO BE IMPLEMENTED IN THIS FDD USED ONLY FOR SIMULATION PURPOSES/1(Qualifier) -> Terminator2/1
  Only here because I could not get model to run with enumerations in the stateflow diagram/1 -> ISO Fault Debounce Design NOT TO BE IMPLEMENTED IN THIS FDD USED ONLY FOR SIMULATION PURPOSES/1(NtcSts)
